simulink model "RigidCompliance"  (R2016a)
settings: Solver=ode4  StartTime=0.0  StopTime=50  FixedStep=0.001  RelTol=1e-3
InitFcn:
  | %%%%%%%%%%%%%%%%%%%%%%%%%%%Controller
  | %Desired position of robot
  | T_des = [-0.3827 0 -0.9239 -0.5134;0 1 0 0;0.9239 0 -0.3827 0.5303;0 0 0 1];
  | %q_d = [0;pi/8;0;-pi/2;0;0;0];
  | 
  | 
  | %Proportional gains of compliance controller
  | K_x = [1500;1500;1500;200;200;200];
  | 
  | %Derivative gains of compliance controller
  | D_x =[500;150;500;20;20;20];
  | 
  | 
  | 
  | %%%%%%%%%%%%%%%%%%%%%%%%%%%Robot's initial
  | %Initial position of robot
  | q_0 = [-0.706;0.4326;0.9182;-1.696;-77.63;-1.726;0.2022];
  | %T_0 = [0.7508 -4063 0.5208 -0.4738;0.3266 -0.457 -0.8273 -8.688e-06;0.5741 0.7913 -0.2104 0.5303;0 0 0 1];
  | %q_0 = [0;0;0;-pi/2;0;0;0];
  | %T_0 = [0 0 -1 -0.39;0 1 0 0;1 0 0 0.71;0 0 0 1]
  | 
  | 
  | 
  | %%%%%%%%%%%%%%%%%%%%%%%%%%%Wall
  | %Parameters of wall plane: ax+by+cz
  | Pl_w = [1;0;0];
  | 
  | %Wall stiffness
  | K_w = [2500;0;0];
  | 
  | %Wall first offset
  | d1 = -0.45;
  | 
  | %Wall second position
  | d2 = -10;
  | 
  | 
  | 
  | %%%%%%%%%%%%%%%%%%%%%%%%%%% Load
  | %Mass of the load
  | m_EE = 0;
  | 
  | %Position of the load
  | rCEE = zeros(3,1);
  | 
  | %T matrix for the load
  | TCP_T_EE = eye(4);
libraries: lwr_dynamics x5
settings Model: Creator=shahriari  LastModifiedBy=shahriari

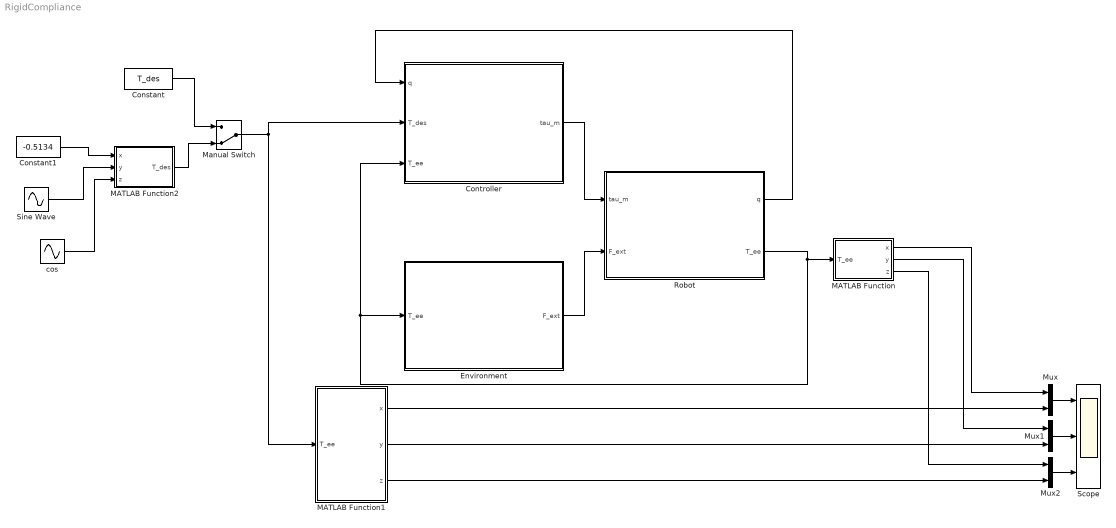
== system RigidCompliance ==
  Constant : Constant  Value=T_des
  Constant1 : Constant  Value=-0.5134
  Controller : Subsystem
  Environment : Subsystem
  MATLAB Function : MATLAB Function  TreatAsAtomicUnit=on
  MATLAB Function1 : MATLAB Function  TreatAsAtomicUnit=on
  MATLAB Function2 : MATLAB Function  TreatAsAtomicUnit=on
  Manual Switch : ManualSwitch  CurrentSetting=0
  Mux : Mux  Inputs=2
  Mux1 : Mux  Inputs=2
  Mux2 : Mux  Inputs=2
  Robot : Subsystem
  Scope : Scope  NumInputPorts=3
  Sine Wave : Sin  Amplitude=0.1492  Frequency=0.01  SampleTime=0
  cos : Sin  Amplitude=-0.1492  Bias=0.6795  Frequency=0.01  Phase=pi/2  SampleTime=0
  wires:
  Controller/1(tau_m) -> Robot/1(tau_m)
  Robot/2(T_ee) -> Controller/3(T_ee), Environment/1(T_ee), MATLAB Function/1(T_ee)
  Environment/1(F_ext) -> Robot/2(F_ext)
  Robot/1(q) -> Controller/1(q)
  Manual Switch/1 -> MATLAB Function1/1(T_ee), Controller/2(T_des)
  Mux/1 -> Scope/1
  Mux1/1 -> Scope/2
  Mux2/1 -> Scope/3
  MATLAB Function/1(x) -> Mux/1
  MATLAB Function1/1(x) -> Mux/2
  MATLAB Function1/2(y) -> Mux1/2
  MATLAB Function1/3(z) -> Mux2/2
  MATLAB Function/2(y) -> Mux1/1
  MATLAB Function/3(z) -> Mux2/1
  MATLAB Function2/1(T_des) -> Manual Switch/2
  Constant/1 -> Manual Switch/1
  Constant1/1 -> MATLAB Function2/1(x)
  Sine Wave/1 -> MATLAB Function2/2(y)
  cos/1 -> MATLAB Function2/3(z)

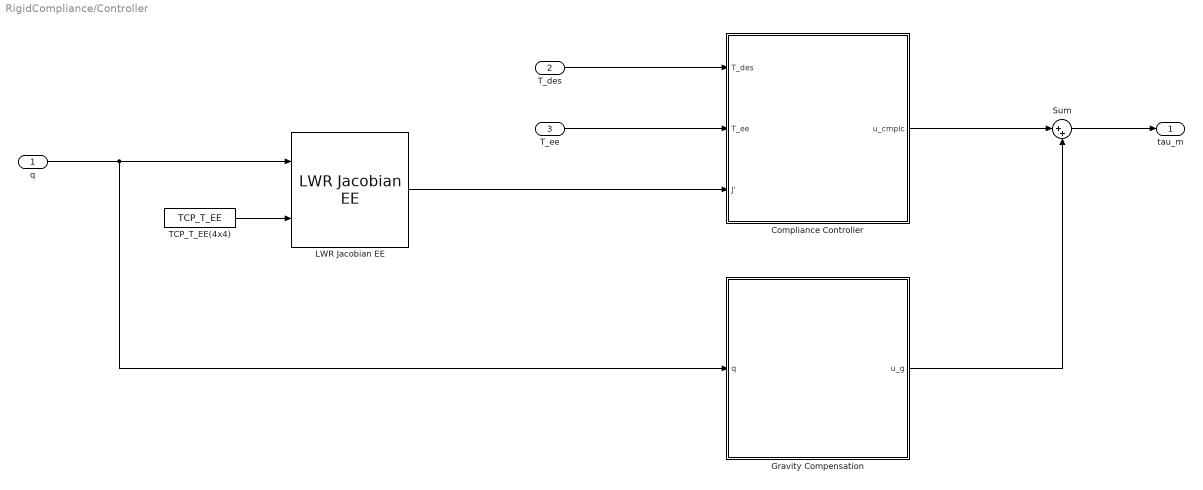
== system RigidCompliance/Controller ==
  q : Inport
  T_des : Inport  Port=2
  T_ee : Inport  Port=3
  Compliance Controller : Subsystem
  Gravity Compensation : Subsystem
  LWR Jacobian EE : lwr_dynamics/Kinematics/LWR Jacobian EE
  Sum : Sum  Inputs=|++
  TCP_T_EE(4x4) : Constant  Value=TCP_T_EE
  tau_m : Outport
  wires:
  Sum/1 -> tau_m/1
  Compliance Controller/1(" u_cmplc") -> Sum/1
  Gravity Compensation/1(u_g) -> Sum/2
  TCP_T_EE(4x4)/1 -> LWR Jacobian EE/2
  q/1 -> Gravity Compensation/1(q), LWR Jacobian EE/1
  LWR Jacobian EE/1 -> Compliance Controller/3(J')
  T_ee/1 -> Compliance Controller/2(T_ee)
  T_des/1 -> Compliance Controller/1(T_des)

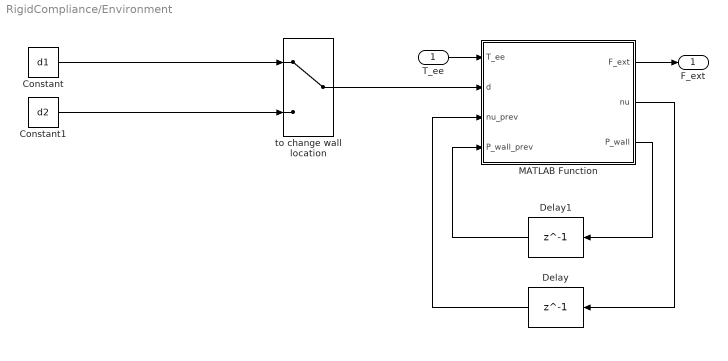
== system RigidCompliance/Environment ==
  T_ee : Inport
  Constant : Constant  Value=d1
  Constant1 : Constant  Value=d2
  Delay : Delay  DelayLength=1  InitialCondition=0  UseCircularBuffer=on
  Delay1 : Delay  DelayLength=1  InitialCondition=zeros(3,1)  UseCircularBuffer=on
  MATLAB Function : MATLAB Function  TreatAsAtomicUnit=on
  to change wall location : ManualSwitch
  F_ext : Outport
  wires:
  to change wall location/1 -> MATLAB Function/2(d)
  Constant/1 -> to change wall location/1
  Constant1/1 -> to change wall location/2
  MATLAB Function/1(F_ext) -> F_ext/1
  MATLAB Function/2(nu) -> Delay/1
  Delay/1 -> MATLAB Function/3(nu_prev)
  MATLAB Function/3(P_wall) -> Delay1/1
  Delay1/1 -> MATLAB Function/4(P_wall_prev)
  T_ee/1 -> MATLAB Function/1(T_ee)

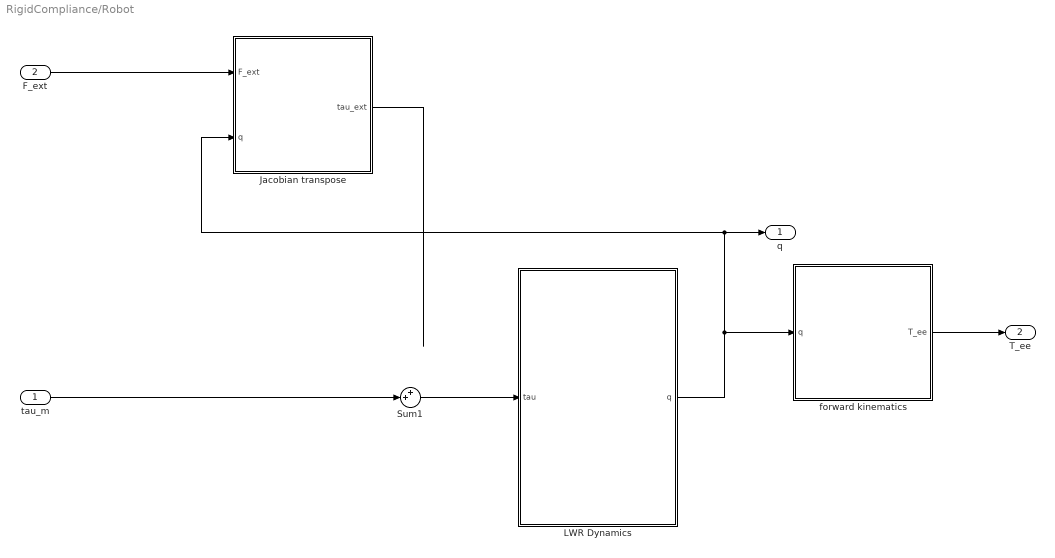
== system RigidCompliance/Robot ==
  tau_m : Inport
  F_ext : Inport  Port=2
  Jacobian transpose : Subsystem
  LWR Dynamics : Subsystem
  Sum1 : Sum  Inputs=++|
  forward kinematics : Subsystem
  q : Outport
  T_ee : Outport  Port=2
  wires:
  Sum1/1 -> LWR Dynamics/1(tau)
  LWR Dynamics/1(q) -> Jacobian transpose/2(q), q/1, forward kinematics/1(q)
  forward kinematics/1("T_ee ") -> T_ee/1
  F_ext/1 -> Jacobian transpose/1(F_ext)
  Jacobian transpose/1(tau_ext) -> ?
  tau_m/1 -> Sum1/2

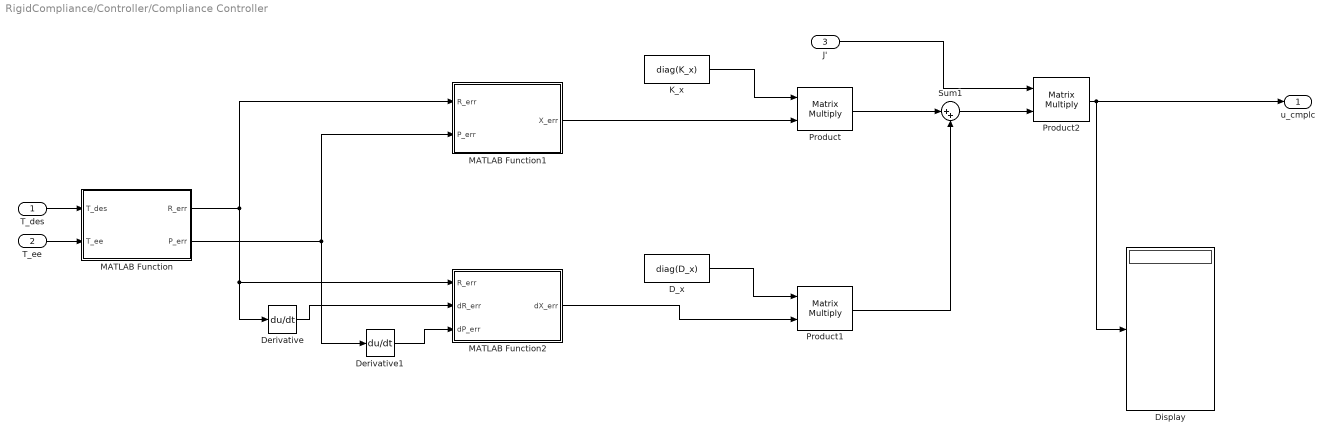
== system RigidCompliance/Controller/Compliance Controller ==
  T_des : Inport
  T_ee : Inport  Port=2
  J' : Inport  Port=3
  D_x : Constant  Value=diag(D_x)
  Derivative : Derivative
  Derivative1 : Derivative
  Display : Display
  K_x : Constant  Value=diag(K_x)
  MATLAB Function : MATLAB Function  TreatAsAtomicUnit=on
  MATLAB Function1 : MATLAB Function  TreatAsAtomicUnit=on
  MATLAB Function2 : MATLAB Function  TreatAsAtomicUnit=on
  Product : Product  Multiplication=Matrix(*)
  Product1 : Product  Multiplication=Matrix(*)
  Product2 : Product  Multiplication=Matrix(*)
  Sum1 : Sum  Inputs=|++
  " u_cmplc" : Outport
  wires:
  K_x/1 -> Product/1
  D_x/1 -> Product1/1
  Product/1 -> Sum1/1
  Product1/1 -> Sum1/2
  Sum1/1 -> Product2/2
  MATLAB Function1/1(X_err) -> Product/2
  J'/1 -> Product2/1
  T_des/1 -> MATLAB Function/1(T_des)
  T_ee/1 -> MATLAB Function/2(T_ee)
  MATLAB Function/1(R_err) -> MATLAB Function1/1(R_err), MATLAB Function2/1(R_err), Derivative/1
  MATLAB Function/2(P_err) -> MATLAB Function1/2(P_err), Derivative1/1
  Derivative/1 -> MATLAB Function2/2(dR_err)
  Derivative1/1 -> MATLAB Function2/3(dP_err)
  MATLAB Function2/1(dX_err) -> Product1/2
  Product2/1 -> Display/1, " u_cmplc"/1

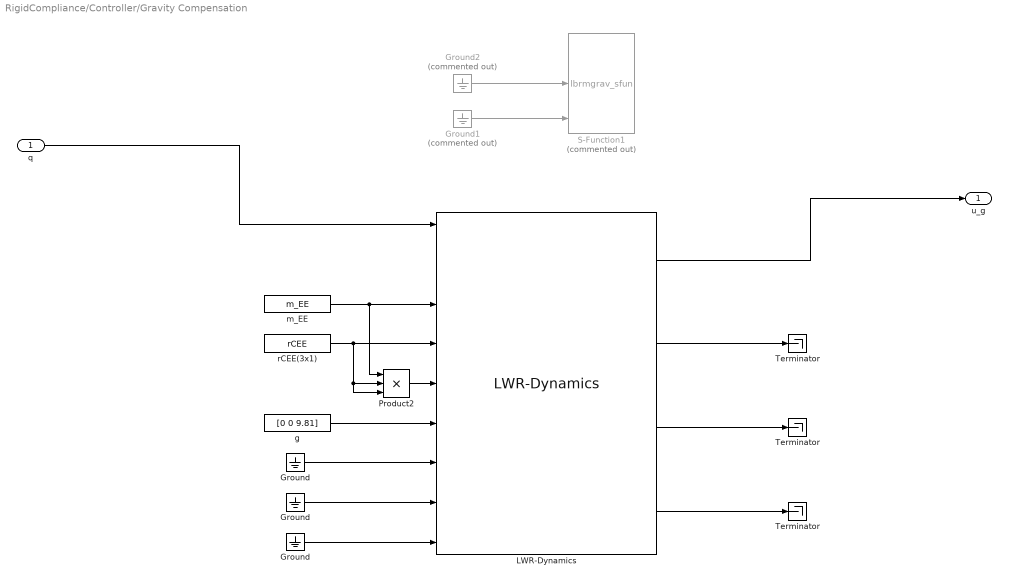
== system RigidCompliance/Controller/Gravity Compensation ==
  q : Inport
  Ground : Ground
  "Ground " : Ground
  "Ground  " : Ground
  Ground1 : Ground  Commented=on
  Ground2 : Ground  Commented=on
  LWR-Dynamics : lwr_dynamics/Dynamics/LWR-Dynamics
  Product2 : Product  Inputs=3  RndMeth=Zero
  S-Function1 : S-Function  Commented=on  FunctionName=lbrmgrav_sfun  SFunctionDeploymentMode=off  EnableBusSupport=off
  Terminator : Terminator
  "Terminator " : Terminator
  "Terminator  " : Terminator
  g : Constant  Value=[0 0 9.81]
  m_EE : Constant  Value=m_EE
  rCEE(3x1) : Constant  Value=rCEE
  u_g : Outport
  wires:
  Ground/1 -> LWR-Dynamics/7
  "Ground "/1 -> LWR-Dynamics/8
  "Ground  "/1 -> LWR-Dynamics/9
  g/1 -> LWR-Dynamics/6
  m_EE/1 -> LWR-Dynamics/3, Product2/1
  rCEE(3x1)/1 -> LWR-Dynamics/4, Product2/3, Product2/2
  Product2/1 -> LWR-Dynamics/5
  LWR-Dynamics/2 -> Terminator/1
  LWR-Dynamics/3 -> "Terminator "/1
  LWR-Dynamics/4 -> "Terminator  "/1
  Ground1/1 -> S-Function1/3
  Ground2/1 -> S-Function1/2
  q/1 -> LWR-Dynamics/1
  LWR-Dynamics/1 -> u_g/1

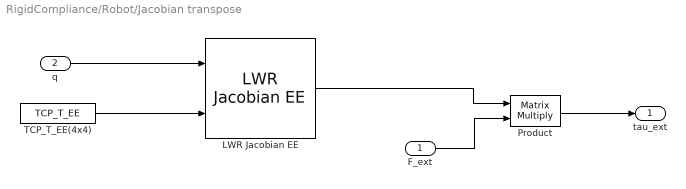
== system RigidCompliance/Robot/Jacobian transpose ==
  F_ext : Inport
  q : Inport  Port=2
  LWR Jacobian EE : lwr_dynamics/Kinematics/LWR Jacobian EE
  Product : Product  Multiplication=Matrix(*)
  TCP_T_EE(4x4) : Constant  Value=TCP_T_EE
  tau_ext : Outport
  wires:
  q/1 -> LWR Jacobian EE/1
  TCP_T_EE(4x4)/1 -> LWR Jacobian EE/2
  Product/1 -> tau_ext/1
  F_ext/1 -> Product/2
  LWR Jacobian EE/1 -> Product/1

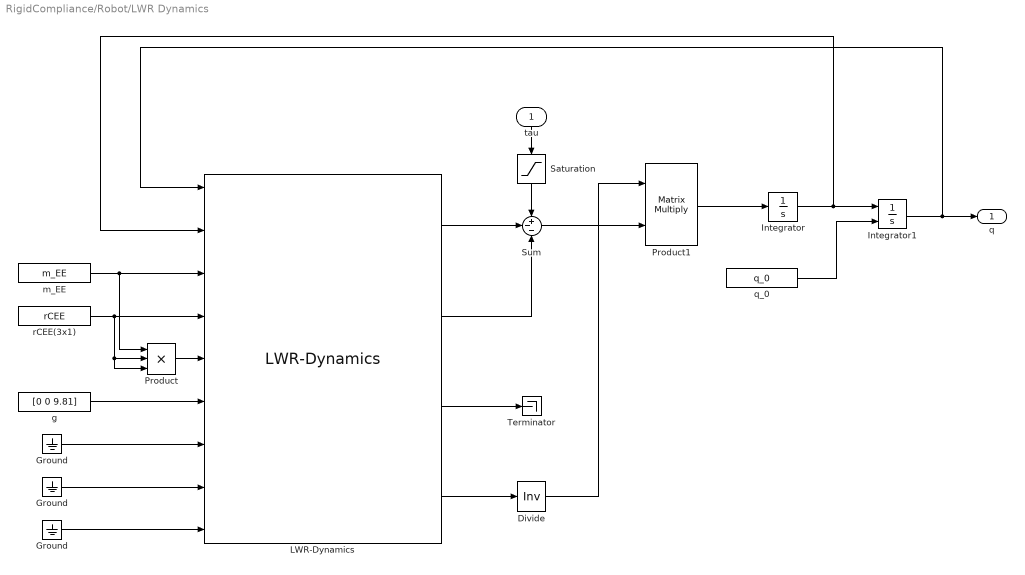
== system RigidCompliance/Robot/LWR Dynamics ==
  tau : Inport
  Divide : Product  Inputs=/  Multiplication=Matrix(*)
  Ground : Ground
  "Ground " : Ground
  "Ground  " : Ground
  Integrator : Integrator  InitialCondition=zeros(7,1)
  Integrator1 : Integrator  InitialConditionSource=external
  LWR-Dynamics : lwr_dynamics/Dynamics/LWR-Dynamics
  Product : Product  Inputs=3  RndMeth=Zero
  Product1 : Product  Multiplication=Matrix(*)  RndMeth=Zero
  Saturation : Saturate  UpperLimit=30  LowerLimit=-30
  Sum : Sum  Inputs=+--
  Terminator : Terminator
  g : Constant  Value=[0 0 9.81]
  m_EE : Constant  Value=m_EE
  q_0 : Constant  Value=q_0
  rCEE(3x1) : Constant  Value=rCEE
  q : Outport
  wires:
  Ground/1 -> LWR-Dynamics/7
  "Ground "/1 -> LWR-Dynamics/8
  "Ground  "/1 -> LWR-Dynamics/9
  g/1 -> LWR-Dynamics/6
  m_EE/1 -> LWR-Dynamics/3, Product/1
  rCEE(3x1)/1 -> LWR-Dynamics/4, Product/3, Product/2
  Product/1 -> LWR-Dynamics/5
  LWR-Dynamics/3 -> Terminator/1
  LWR-Dynamics/4 -> Divide/1
  LWR-Dynamics/1 -> Sum/2
  LWR-Dynamics/2 -> Sum/3
  tau/1 -> Saturation/1
  Product1/1 -> Integrator/1
  Integrator/1 -> LWR-Dynamics/2, Integrator1/1
  q_0/1 -> Integrator1/2
  Integrator1/1 -> LWR-Dynamics/1, q/1
  Sum/1 -> Product1/2
  Divide/1 -> Product1/1
  Saturation/1 -> Sum/1

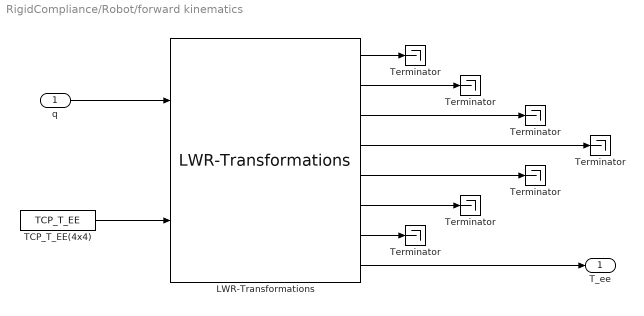
== system RigidCompliance/Robot/forward kinematics ==
  q : Inport
  LWR-Transformations : lwr_dynamics/Kinematics/LWR-Transformations
  TCP_T_EE(4x4) : Constant  Value=TCP_T_EE
  Terminator : Terminator
  "Terminator " : Terminator
  "Terminator  " : Terminator
  "Terminator   " : Terminator
  "Terminator    " : Terminator
  "Terminator     " : Terminator
  "Terminator      " : Terminator
  "T_ee " : Outport
  wires:
  TCP_T_EE(4x4)/1 -> LWR-Transformations/2
  q/1 -> LWR-Transformations/1
  LWR-Transformations/8 -> "T_ee "/1
  LWR-Transformations/1 -> Terminator/1
  LWR-Transformations/2 -> "Terminator "/1
  LWR-Transformations/3 -> "Terminator  "/1
  LWR-Transformations/4 -> "Terminator   "/1
  LWR-Transformations/5 -> "Terminator    "/1
  LWR-Transformations/6 -> "Terminator     "/1
  LWR-Transformations/7 -> "Terminator      "/1

== matlab function RigidCompliance/Environment/MATLAB Function ==
  data: T_ee input; F_ext output; d input; Pl_w parameter; K_w parameter; nu_prev input; nu output; P_wall_prev input; P_wall output
function [F_ext,nu,P_wall] = fcn(T_ee,d, Pl_w, K_w, nu_prev, P_wall_prev)
%#codegen

P_ee = T_ee(1:3,4);


if abs(Pl_w'*P_ee) < abs(d)
    nu = 0;
    P_wall = zeros(3,1);
    F_ext = zeros(6,1);
elseif nu_prev == 0
    nu = 1;
    P_wall = P_ee;
    F_ext = zeros(6,1);
else P_wall = P_wall_prev;
     F_ext = abs([diag(K_w)*(P_ee-P_wall);zeros(3,1)]);
     nu = 1;
end

== matlab function RigidCompliance/Controller/Compliance Controller/MATLAB Function ==
  data: T_des input; R_err output; T_ee input; P_err output
function [R_err, P_err] = fcn(T_des,T_ee)
%#codegen

R_err = T_ee(1:3,1:3)'*T_des(1:3,1:3);
P_err = T_des(1:3,4)-T_ee(1:3,4);

== matlab function RigidCompliance/Controller/Compliance Controller/MATLAB Function1 ==
  data: R_err input; X_err output; P_err input
function X_err  = fcn(R_err, P_err)
%#codegen

X_err = [P_err;zeros(3,1)];%rotm2eul(R_err)'];

== matlab function RigidCompliance/Controller/Compliance Controller/MATLAB Function2 ==
  data: R_err input; dX_err output; dR_err input; dP_err input
function dX_err  = fcn(R_err, dR_err, dP_err)
%#codegen

omega_str_err = dR_err*R_err';
dX_err = [dP_err;zeros(3,1)];%-omega_str_err(2,3);omega_str_err(1,3);-omega_str_err(1,2)];

== matlab function RigidCompliance/MATLAB Function ==
  data: x output; T_ee input; y output; z output
function [x, y, z] = fcn(T_ee)
%#codegen

x = T_ee(1,4);
y = T_ee(2,4);
z = T_ee(3,4);

== matlab function RigidCompliance/MATLAB Function1 ==
  data: x output; T_ee input; y output; z output
function [x, y, z] = fcn(T_ee)
%#codegen

x = T_ee(1,4);
y = T_ee(2,4);
z = T_ee(3,4);

== matlab function RigidCompliance/MATLAB Function2 ==
  data: x input; T_des output; y input; z input
function T_des = fcn(x,y,z)
%#codegen

T_des = [1 0 0 x;0 1 0 y;0 0 1 z;0 0 0 1];
